simulink model "Transformada_de_Park_directa"  (R2021a)
settings: Solver=VariableStepAuto  StartTime=0.0  StopTime=10.0  RelTol=1e-3
settings Model: Creator=fhlla  LastModifiedBy=fhlla

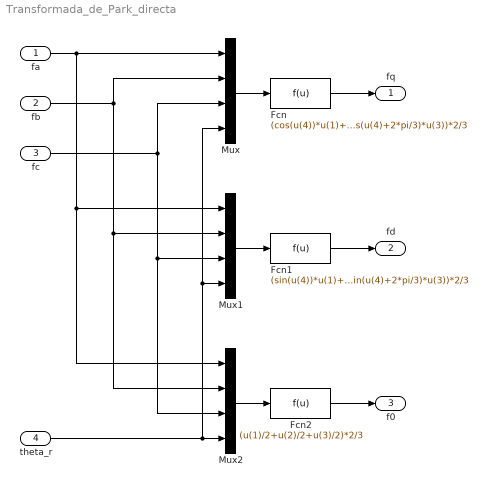
== system Transformada_de_Park_directa ==
  "fa " : Inport
  "fb " : Inport  Port=2
  "fc " : Inport  Port=3
  theta_r : Inport  Port=4
  Fcn : Fcn  Expr=(cos(u(4))*u(1)+cos(u(4)-2*pi/3)*u(2)+cos(u(4)+2*pi/3)*u(3))*2/3
  Fcn1 : Fcn  Expr=(sin(u(4))*u(1)+sin(u(4)-2*pi/3)*u(2)+sin(u(4)+2*pi/3)*u(3))*2/3
  Fcn2 : Fcn  Expr=(u(1)/2+u(2)/2+u(3)/2)*2/3
  Mux : Mux
  Mux1 : Mux
  Mux2 : Mux
  fq : Outport
  fd : Outport  Port=2
  f0 : Outport  Port=3
  wires:
  Mux2/1 -> Fcn2/1
  "fb "/1 -> Mux1/2, Mux2/2, Mux/2
  Fcn1/1 -> fd/1
  theta_r/1 -> Mux/4, Mux1/4, Mux2/4
  "fa "/1 -> Mux/1, Mux1/1, Mux2/1
  Fcn/1 -> fq/1
  Mux1/1 -> Fcn1/1
  Fcn2/1 -> f0/1
  Mux/1 -> Fcn/1
  "fc "/1 -> Mux1/3, Mux2/3, Mux/3
